simulink model "SF044A_HowDetn"  (R2013b)
settings: Solver=FixedStepDiscrete  SolverMode=SingleTasking  StartTime=0.0  StopTime=1  FixedStep=0.002  RelTol=1e-3
values from neighbouring files (symbols this model uses):
  ABSLTHIFRQTQHILIM_HWNWTMTR_F32 = DataDict.Constant    [SF044A_HowDetn_DataDict.m]
  ABSLTHIFRQTQLOLIM_HWNWTMTR_F32 = DataDict.Constant    [SF044A_HowDetn_DataDict.m]
  ARCHGLBPRM_2MILLISEC_SEC_F32 = DataDict.Constant    [SF044A_HowDetn_DataDict.m]
  HOWDETNESTIMNLIM_ULS_F32 = DataDict.Constant    [SF044A_HowDetn_DataDict.m]
  HOWDETNESTIMNTHD_ULS_F32 = DataDict.Constant    [SF044A_HowDetn_DataDict.m]
  HowDetnHiFrqGainY = DataDict.Calibration    [SF044A_HowDetn_DataDict.m]
  HowDetnMinVehSpd = DataDict.Calibration    [SF044A_HowDetn_DataDict.m]
  HowDetnPercOfPrevHowEstim = DataDict.Calibration    [SF044A_HowDetn_DataDict.m]
  HowDetnSlewRate = DataDict.Calibration    [SF044A_HowDetn_DataDict.m]
  HowDetnVehSpd = DataDict.Calibration    [SF044A_HowDetn_DataDict.m]
libraries: Fil x14, FloatToFixd x6, NxtrLim x5, FixdToFloat x3, BilnrIntrpnMplX x2, NxtrAbslt x2, simulink x2, LnrIntrpn x1, LnrIntrpnDyn x1
(part 2 of 2)

== system SF044A_HowDetn/HowDetn/HowDetnPer1/Calculate HOW Estimate/Low-Frequency Lookup Table/CopyRight2 ==

== system SF044A_HowDetn/HowDetn/HowDetnPer1/Calculate HOW Estimate/default/CopyRight2 ==

== system SF044A_HowDetn/HowDetn/HowDetnPer1/Determine HOW State/HOW State Look up Table/CopyRight2 ==

== system SF044A_HowDetn/HowDetn/HowDetnPer1/Determine HOW State/Pass/CopyRight2 ==

== system SF044A_HowDetn/HowDetn/HowDetnPer1/Determine HOW State/Zero/CopyRight2 ==
